simulink library "fdclib5"  (Simulink 3.00)
undefined symbols (not defined in the file): AM, GM1, GM2, xfix, xinco
libraries: fdclib5 x7, simulink3 x1
settings Model: LastModifiedBy=Dutchroll

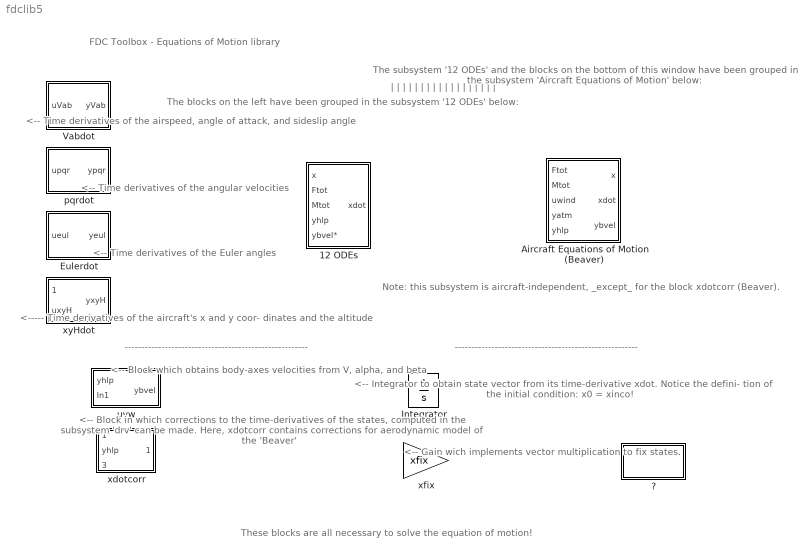
== system fdclib5 ==
  note: <-- Block which obtains body-axes
      | velocities from V, alpha, and beta
  note: <-- Block in which corrections to the
      | time-derivatives of the states, computed
      | in the subsystem 'drv' can be made.
      | Here, xdotcorr contains corrections for
      | aerodynamic model of the 'Beaver'
  note: <-- Gain wich implements vector
      | multiplication to fix states.
  note: <-- Integrator to obtain state vector from
      | its time-derivative xdot. Notice the defini-
      | tion of the initial condition: x0 = xinco!
  note: |
      | |
      | |
      | |
      | |
      | |
      | |
      | |
      | |
      | |
      | |
      | |
      | |
      | |
      | |
      | |
      | |
      | |
  note: The blocks on the left have
      | been grouped in the
      | subsystem '12 ODEs' below:
  note: The subsystem '12 ODEs' and the
      | blocks on the bottom of this window
      | have been grouped in the subsystem
      | 'Aircraft Equations of Motion' below:
  note: FDC Toolbox - Equations of Motion library
  note: -------------------------------------------------------
  note: <-----  Time derivatives of
      | the aircraft's x and y coor-
      | dinates and the altitude
  note: <-- Time derivatives of
      | the Euler angles
  note: <-- Time derivatives of
      | the angular velocities
  note: <-- Time derivatives of
      | the airspeed, angle of
      | attack, and sideslip angle
  note: -------------------------------------------------------
  note: Note: this subsystem is aircraft-independent,
      |  _except_ for the block xdotcorr (Beaver).
  note: These blocks are all necessary to solve the equation of motion!
  12 ODEs : Subsystem
  "?" : Subsystem
      settings: OpenFcn=browse xfix
      mask Display: disp('More info\nabout xfix')
  Aircraft Equations of Motion (Beaver) : Subsystem
  Eulerdot : Subsystem
      mask Type: Eulerdot
      mask Description:
      | Calculation of d(psi)/dt, d(theta)/dt,
      | and d(phi/dt)
      mask Help: eval('browse eulerdot')
      mask Display: disp('psi dot\ntheta dot\nphi dot')
  Integrator : Integrator  ExternalReset=none  InitialConditionSource=internal  InitialCondition=xinco  LimitOutput=off  UpperSaturationLimit=inf  LowerSaturationLimit=-inf  ShowSaturationPort=off  ShowStatePort=off  AbsoluteTolerance=auto
  Vabdot : Subsystem  mask(Vabdot){m=GM1(10)}
      mask prompts: m "Mass of the aircraft [kg]:"
      mask help: Calculation of dV/dt, dalpha/dt, dbeta/dt.
      mask Help: eval('browse vabdot')
      mask Display: disp('V dot\nalpha dot\nbeta dot')
  pqrdot : Subsystem
      mask Type: pqrdot
      mask Description: Calculation of dp/dt, dq/dt, and dr/dt
      mask Help: eval('browse pqrdot')
      mask Display: disp('p dot\nq dot\nr dot')
  uvw : Subsystem
      mask Type: uvw
      mask Description:
      | Calculation of body-axes velocities
      | u, v, and w
      mask Help: eval('browse uvw')
      mask Display: disp('Body-axes\nvelocities')
  xdotcorr : Subsystem  mask(xdotcorr){b=GM1(2), S=GM1(3), m=GM1(10), CYbdot=AM(2,19)}
      mask prompts: b "Wing span [m]:"; S "Wing surface [m^2]:"; m "Mass of the aircraft [kg]:"; CYbdot "Stability-derivative CYbdot:"
      mask help:
      | Correction block to write state
      | equations for DHC-2 Beaver aircraft
      | explicitly.
      mask Help: eval('browse xdotcorr')
      mask Display: disp('xdotcorr\n(Beaver)')
  xfix : Gain  InitFcn=if exist('xfix')==0, xfix=ones(12,1); end  Gain=xfix  SaturateOnIntegerOverflow=on
  xyHdot : Subsystem
      mask Type: xyHdot
      mask Description: Calculation of d(xe)/dt, d(ye)/dt, and dH/dt
      mask Help: eval('browse xyhdot')
      mask Display: disp('xe dot\nye dot\nH dot')

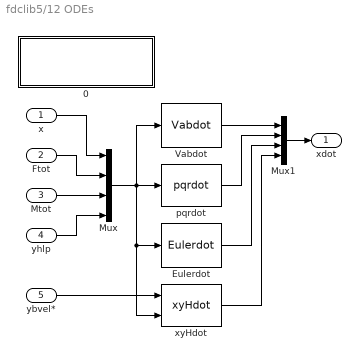
== system fdclib5/12 ODEs ==
  x : Inport  Port=1  PortWidth=-1  SampleTime=-1  DataType=auto
      settings: SignalType=auto
  Ftot : Inport  Port=2  PortWidth=-1  SampleTime=-1  DataType=auto
      settings: SignalType=auto
  Mtot : Inport  Port=3  PortWidth=-1  SampleTime=-1  DataType=auto
      settings: SignalType=auto
  yhlp : Inport  Port=4  PortWidth=-1  SampleTime=-1  DataType=auto
      settings: SignalType=auto
  ybvel* : Inport  Port=5  PortWidth=-1  SampleTime=-1  DataType=auto
      settings: SignalType=auto
  0 : Subsystem
      settings: OpenFcn=browse 12odes
      mask Display: disp('12 Ordinary Differential\nEquations (level 4)\nM.O. Rauw')
  Eulerdot : fdclib5/Eulerdot
  Mux : Mux  Inputs=[12 3 3 11]
      settings: DisplayOption=none
  Mux1 : Mux  Inputs=[3 3 3 3]
      settings: DisplayOption=none
  Vabdot : fdclib5/Vabdot  m=GM1(10)
  pqrdot : fdclib5/pqrdot
  xyHdot : fdclib5/xyHdot
  xdot : Outport  Port=1
  wires:
  Mux1/1 -> xdot/1
  Vabdot/1 -> Mux1/1
  pqrdot/1 -> Mux1/2
  Eulerdot/1 -> Mux1/3
  xyHdot/1 -> Mux1/4
  yhlp/1 -> Mux/4
  ybvel*/1 -> xyHdot/1
  Mux/1 -> xyHdot/2, Eulerdot/1, Vabdot/1, pqrdot/1
  Ftot/1 -> Mux/2
  Mtot/1 -> Mux/3
  x/1 -> Mux/1

== system fdclib5/? ==

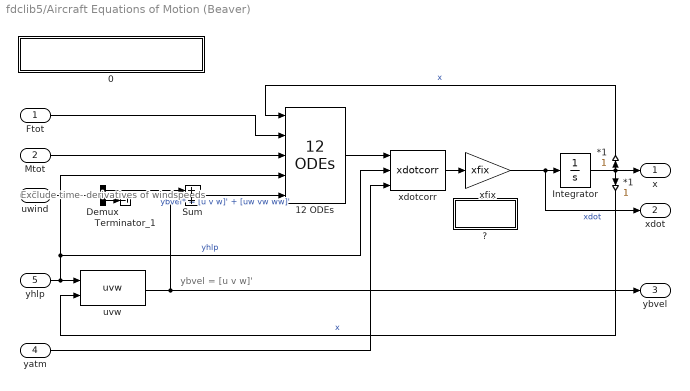
== system fdclib5/Aircraft Equations of Motion (Beaver) ==
  note: ybvel = [u v w]'
  note: Exclude time-
      | derivatives
      | of windspeeds
  Ftot : Inport  Port=1  PortWidth=-1  SampleTime=-1  DataType=auto
      settings: SignalType=auto
  Mtot : Inport  Port=2  PortWidth=-1  SampleTime=-1  DataType=auto
      settings: SignalType=auto
  uwind : Inport  Port=3  PortWidth=-1  SampleTime=-1  DataType=auto
      settings: SignalType=auto
  yatm : Inport  Port=4  PortWidth=-1  SampleTime=-1  DataType=auto
      settings: SignalType=auto
  yhlp : Inport  Port=5  PortWidth=-1  SampleTime=-1  DataType=auto
      settings: SignalType=auto
  " *1" : Gain  Orientation=up  Gain=1  SaturateOnIntegerOverflow=on
  *1 : Gain  Orientation=down  Gain=1  SaturateOnIntegerOverflow=on
  0 : Subsystem
      settings: OpenFcn=browse eqmotion
      mask Display: disp('EQUATIONS OF MOTION (level 3)\nM.O. Rauw')
  12 ODEs : fdclib5/12 ODEs
  "?" : Subsystem
      settings: OpenFcn=browse xfix
      mask Display: disp('More info\nfor xfix')
  Demux : Demux  Outputs=[3 3]
  Integrator : Integrator  ExternalReset=none  InitialConditionSource=internal  InitialCondition=xinco  LimitOutput=off  UpperSaturationLimit=inf  LowerSaturationLimit=-inf  ShowSaturationPort=off  ShowStatePort=off  AbsoluteTolerance=auto
  Sum : Sum  Inputs=++  SaturateOnIntegerOverflow=on
  Terminator_1 : Terminator
  uvw : fdclib5/uvw
  xdotcorr : fdclib5/xdotcorr  b=GM1(2)  S=GM1(3)  m=GM1(10)  CYbdot=AM(2,19)
  xfix : Gain  InitFcn=if exist('xfix')==0, xfix=ones(12,1); end  Gain=xfix  SaturateOnIntegerOverflow=on
  x : Outport  Port=1
  xdot : Outport  Port=2
  ybvel : Outport  Port=3
  wires:
  yhlp/1 -> uvw/1, 12 ODEs/4, xdotcorr/2  "yhlp"
  Sum/1 -> 12 ODEs/5  "ybvel* = [u v w]' + [uw vw ww]'"
  uvw/1 -> ybvel/1, Sum/2
  uwind/1 -> Demux/1
  Demux/1 -> Sum/1
  Ftot/1 -> 12 ODEs/2
  Mtot/1 -> 12 ODEs/3
  12 ODEs/1 -> xdotcorr/1
  xdotcorr/1 -> xfix/1
  yatm/1 -> xdotcorr/3
  *1/1 -> uvw/2  "x"
  xfix/1 -> Integrator/1, xdot/1  "xdot"
  " *1"/1 -> 12 ODEs/1  "x"
  Demux/2 -> Terminator_1/1
  Integrator/1 -> x/1, " *1"/1, *1/1

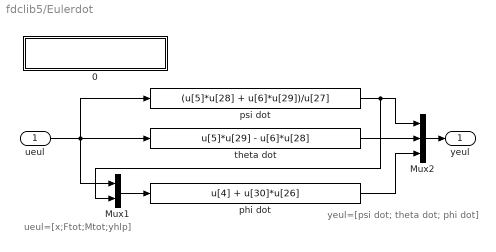
== system fdclib5/Eulerdot ==
  note: yeul=[psi dot; theta dot; phi dot]
  note: ueul=[x;Ftot;Mtot;yhlp]
  ueul : Inport  Port=1  PortWidth=-1  SampleTime=-1  DataType=auto
      settings: SignalType=auto
  0 : Subsystem
      settings: OpenFcn=browse eulerdot
      mask Display: disp('EULERDOT\nM.O. Rauw, March 2003')
  Mux1 : Mux  Inputs=[29 1]
      settings: DisplayOption=none
  Mux2 : Mux  Inputs=3
      settings: DisplayOption=none
  phi dot : Fcn  Expr=u[4] + u[30]*u[26]
  psi dot : Fcn  Expr=(u[5]*u[28] + u[6]*u[29])/u[27]
  theta dot : Fcn  Expr=u[5]*u[29] - u[6]*u[28]
  yeul : Outport  Port=1
  wires:
  Mux1/1 -> phi dot/1
  phi dot/1 -> Mux2/3
  Mux2/1 -> yeul/1
  theta dot/1 -> Mux2/2
  psi dot/1 -> Mux1/2, Mux2/1
  ueul/1 -> psi dot/1, Mux1/1, theta dot/1

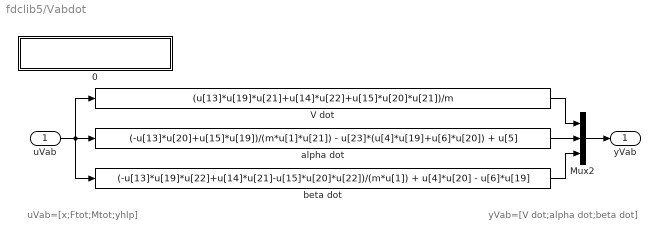
== system fdclib5/Vabdot ==
  note: uVab=[x;Ftot;Mtot;yhlp]
  note: yVab=[V dot;alpha dot;beta dot]
  uVab : Inport  Port=1  PortWidth=-1  SampleTime=-1  DataType=auto
      settings: SignalType=auto
  0 : Subsystem
      settings: OpenFcn=browse vabdot
      mask Display: disp('VABDOT\nM.O. Rauw, March 2003')
  Mux2 : Mux  Inputs=3
      settings: DisplayOption=none
  V dot : Fcn  Expr=(u[13]*u[19]*u[21]+u[14]*u[22]+u[15]*u[20]*u[21])/m
  alpha dot : Fcn  Expr=(-u[13]*u[20]+u[15]*u[19])/(m*u[1]*u[21]) - u[23]*(u[4]*u[19]+u[6]*u[20]) + u[5]
  beta dot : Fcn  Expr=(-u[13]*u[19]*u[22]+u[14]*u[21]-u[15]*u[20]*u[22])/(m*u[1]) + u[4]*u[20] - u[6]*u[19]
  yVab : Outport  Port=1
  wires:
  Mux2/1 -> yVab/1
  uVab/1 -> V dot/1, beta dot/1, alpha dot/1
  alpha dot/1 -> Mux2/2
  V dot/1 -> Mux2/1
  beta dot/1 -> Mux2/3

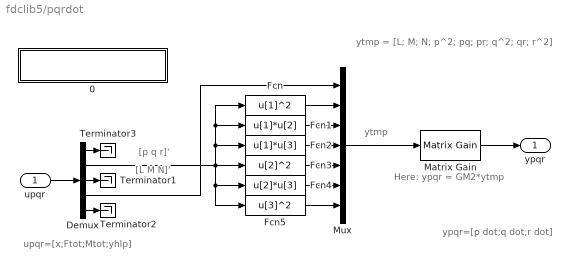
== system fdclib5/pqrdot ==
  note: [p q r]'
  note: [L M N]'
  note: Here: ypqr = GM2*ytmp
  note: ytmp
  note: ypqr=[p dot;q dot;r dot]
  note: upqr=[x;Ftot;Mtot;yhlp]
  note: ytmp = [L; M; N; p^2; pq; pr; q^2; qr; r^2]
  upqr : Inport  Port=1  PortWidth=-1  SampleTime=-1  DataType=auto
      settings: SignalType=auto
  0 : Subsystem
      settings: OpenFcn=browse pqrdot
      mask Display: disp('PQRDOT\nM.O. Rauw, March 2003')
  Demux : Demux  Outputs=[3 3 9 3 11]
  Fcn : Fcn  Expr=u[1]^2
  Fcn1 : Fcn  Expr=u[1]*u[2]
  Fcn2 : Fcn  Expr=u[1]*u[3]
  Fcn3 : Fcn  Expr=u[2]^2
  Fcn4 : Fcn  Expr=u[2]*u[3]
  Fcn5 : Fcn  Expr=u[3]^2
  Matrix Gain : simulink3/Math/Matrix Gain  K=GM2
  Mux : Mux  Inputs=[3 1 1 1 1 1 1]
      settings: DisplayOption=none
  Terminator1 : Terminator
  Terminator2 : Terminator
  Terminator3 : Terminator
  ypqr : Outport  Port=1
  wires:
  Fcn/1 -> Mux/2
  Fcn1/1 -> Mux/3
  Fcn2/1 -> Mux/4
  Fcn3/1 -> Mux/5
  Fcn4/1 -> Mux/6
  Fcn5/1 -> Mux/7
  Matrix Gain/1 -> ypqr/1
  Mux/1 -> Matrix Gain/1
  upqr/1 -> Demux/1
  Demux/1 -> Terminator3/1
  Demux/5 -> Terminator2/1
  Demux/3 -> Terminator1/1
  Demux/2 -> Fcn1/1, Fcn/1, Fcn2/1, Fcn4/1, Fcn5/1, Fcn3/1
  Demux/4 -> Mux/1

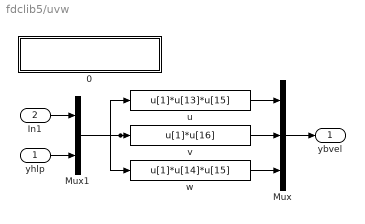
== system fdclib5/uvw ==
  yhlp : Inport  Port=1  PortWidth=-1  SampleTime=-1  DataType=auto
      settings: SignalType=auto
  In1 : Inport  Port=2  PortWidth=-1  SampleTime=-1  DataType=auto
      settings: SignalType=auto
  0 : Subsystem
      settings: OpenFcn=browse uvw
      mask Display: disp('UVW\nM.O. Rauw, March 2003')
  Mux : Mux  Inputs=3
      settings: DisplayOption=none
  Mux1 : Mux  Inputs=[12 11]
      settings: DisplayOption=none
  u : Fcn  Expr=u[1]*u[13]*u[15]
  v : Fcn  Expr=u[1]*u[16]
  w : Fcn  Expr=u[1]*u[14]*u[15]
  ybvel : Outport  Port=1
  wires:
  Mux/1 -> ybvel/1
  w/1 -> Mux/3
  v/1 -> Mux/2
  u/1 -> Mux/1
  In1/1 -> Mux1/1
  yhlp/1 -> Mux1/2
  Mux1/1 -> w/1, u/1, v/1

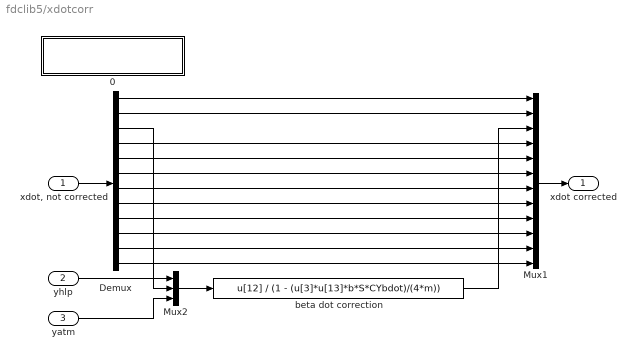
== system fdclib5/xdotcorr ==
  "xdot, not corrected " : Inport  Port=1  PortWidth=-1  SampleTime=-1  DataType=auto
      settings: SignalType=auto
  yhlp : Inport  Port=2  PortWidth=-1  SampleTime=-1  DataType=auto
      settings: SignalType=auto
  yatm : Inport  Port=3  PortWidth=-1  SampleTime=-1  DataType=auto
      settings: SignalType=auto
  0 : Subsystem
      settings: OpenFcn=browse xdotcorr
      mask Display: disp('XDOTCORR (Beaver)\nM.O. Rauw, March 2003')
  Demux : Demux  Outputs=12
  Mux1 : Mux  Inputs=12
      settings: DisplayOption=none
  Mux2 : Mux  Inputs=[11 1 5]
      settings: DisplayOption=none
  beta dot correction : Fcn  Expr=u[12] / (1 - (u[3]*u[13]*b*S*CYbdot)/(4*m))
  xdot corrected : Outport  Port=1
  wires:
  yhlp/1 -> Mux2/1
  Mux2/1 -> beta dot correction/1
  Mux1/1 -> xdot corrected/1
  "xdot, not corrected "/1 -> Demux/1
  Demux/3 -> Mux2/2
  Demux/12 -> Mux1/12
  Demux/11 -> Mux1/11
  Demux/10 -> Mux1/10
  Demux/9 -> Mux1/9
  Demux/8 -> Mux1/8
  Demux/7 -> Mux1/7
  Demux/6 -> Mux1/6
  Demux/5 -> Mux1/5
  Demux/4 -> Mux1/4
  Demux/2 -> Mux1/2
  Demux/1 -> Mux1/1
  yatm/1 -> Mux2/3
  beta dot correction/1 -> Mux1/3

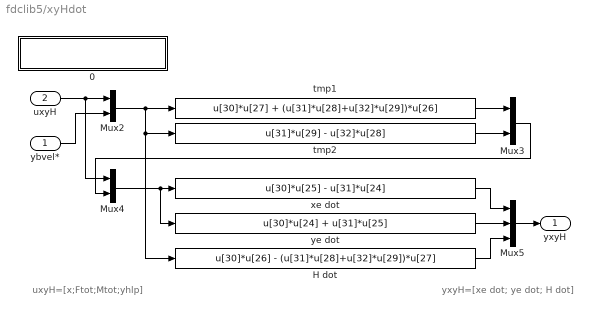
== system fdclib5/xyHdot ==
  note: yxyH=[xe dot; ye dot; H dot]
  note: uxyH=[x;Ftot;Mtot;yhlp]
  ybvel* : Inport  Port=1  PortWidth=-1  SampleTime=-1  DataType=auto
      settings: SignalType=auto
  uxyH : Inport  Port=2  PortWidth=-1  SampleTime=-1  DataType=auto
      settings: SignalType=auto
  0 : Subsystem
      settings: OpenFcn=browse xyhdot
      mask Display: disp('XYHDOT\nM.O. Rauw, March 2003')
  H dot : Fcn  Expr=u[30]*u[26] - (u[31]*u[28]+u[32]*u[29])*u[27]
  Mux2 : Mux  Inputs=[29 3]
      settings: DisplayOption=none
  Mux3 : Mux  Inputs=2
      settings: DisplayOption=none
  Mux4 : Mux  Inputs=[29 2]
      settings: DisplayOption=none
  Mux5 : Mux  Inputs=3
      settings: DisplayOption=none
  tmp1 : Fcn  Expr=u[30]*u[27] + (u[31]*u[28]+u[32]*u[29])*u[26]
  tmp2 : Fcn  Expr=u[31]*u[29] - u[32]*u[28]
  xe dot : Fcn  Expr=u[30]*u[25] - u[31]*u[24]
  ye dot : Fcn  Expr=u[30]*u[24] + u[31]*u[25]
  yxyH : Outport  Port=1
  wires:
  tmp1/1 -> Mux3/1
  H dot/1 -> Mux5/3
  xe dot/1 -> Mux5/1
  tmp2/1 -> Mux3/2
  ye dot/1 -> Mux5/2
  Mux5/1 -> yxyH/1
  Mux4/1 -> ye dot/1, xe dot/1
  Mux2/1 -> H dot/1, tmp2/1, tmp1/1
  Mux3/1 -> Mux4/2
  ybvel*/1 -> Mux2/2
  uxyH/1 -> Mux4/1, Mux2/1

== system fdclib5/12 ODEs/0 ==

== system fdclib5/Aircraft Equations of Motion (Beaver)/0 ==

== system fdclib5/Aircraft Equations of Motion (Beaver)/? ==

== system fdclib5/Eulerdot/0 ==

== system fdclib5/Vabdot/0 ==

== system fdclib5/pqrdot/0 ==

== system fdclib5/uvw/0 ==

== system fdclib5/xdotcorr/0 ==

== system fdclib5/xyHdot/0 ==
